simulink model "step_NL"  (R2023a)
settings: Solver=VariableStepAuto  StartTime=0.0  StopTime=70  RelTol=1e-3
values from neighbouring files (symbols this model uses):
  Ad = 60    [Script_Dirigibile.m]
  b = 20    [Script_Dirigibile.m]
  c = 12.5    [Script_Dirigibile.m]
  Cd = 0.05    [Script_Dirigibile.m]
  g = 9.81    [Script_Dirigibile.m]
  k = 15    [Script_Dirigibile.m]
  m = 1000    [Script_Dirigibile.m]
  rho_a = 1.225    [Script_Dirigibile.m]
  T_a = 288.15    [Script_Dirigibile.m]
  V = 4000    [Script_Dirigibile.m]
  x0 = [0 0 T_a]'    [Script_Dirigibile.m]
settings Model: Creator=giuco  LastModifiedBy=giuco

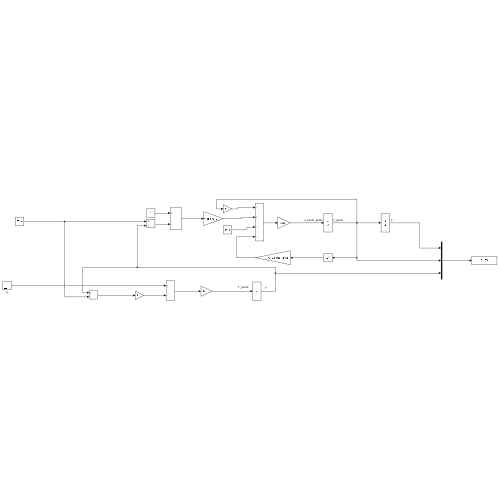
[thumbnail: Simulink's stored preview of the top-level diagram]
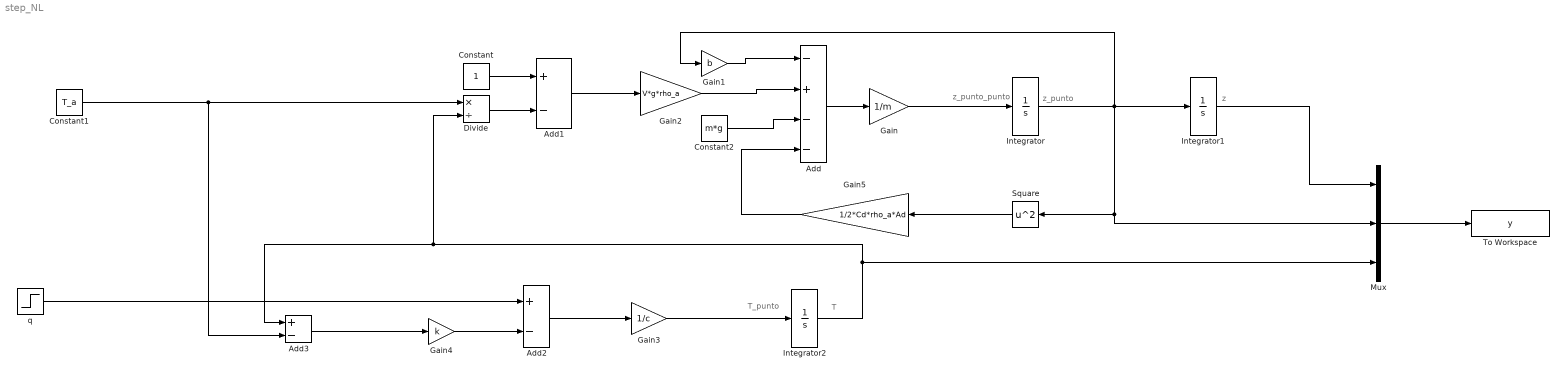
== system step_NL ==
  note: z_punto
  note: T_punto
  note: z
  note: T
  note: z_punto_punto
  Add : Sum  Inputs=-+--
  Add1 : Sum  Inputs=+-
  Add2 : Sum  Inputs=+-
  Add3 : Sum  Inputs=+-
  Constant : Constant
  Constant1 : Constant  Value=T_a
  Constant2 : Constant  Value=m*g
  Divide : Product  Inputs=*/
  Gain : Gain  Gain=1/m
  Gain1 : Gain  Gain=b
  Gain2 : Gain  Gain=V*g*rho_a
  Gain3 : Gain  Gain=1/c
  Gain4 : Gain  Gain=k
  Gain5 : Gain  Gain=1/2*Cd*rho_a*Ad
  Integrator : Integrator  InitialCondition=x0(2)
  Integrator1 : Integrator  InitialCondition=x0(1)
  Integrator2 : Integrator  InitialCondition=x0(3)
  Mux : Mux  Inputs=3
  Square : Math  Operator=square
  To Workspace : ToWorkspace  VariableName=y  SaveFormat=Timeseries  SampleTime=-1
  q : Step  Time=0  After=1500  SampleTime=0
  wires:
  Add1/1 -> Gain2/1
  q/1 -> Add2/1
  Square/1 -> Gain5/1
  Integrator1/1 -> Mux/1
  Gain2/1 -> Add/2
  Mux/1 -> To Workspace/1
  Gain3/1 -> Integrator2/1
  Constant/1 -> Add1/1
  Constant1/1 -> Add3/2, Divide/1
  Gain5/1 -> Add/4
  Add3/1 -> Gain4/1
  Integrator2/1 -> Mux/3, Add3/1, Divide/2
  Gain1/1 -> Add/1
  Divide/1 -> Add1/2
  Gain4/1 -> Add2/2
  Integrator/1 -> Square/1, Mux/2, Gain1/1, Integrator1/1
  Add2/1 -> Gain3/1
  Constant2/1 -> Add/3
  Add/1 -> Gain/1
  Gain/1 -> Integrator/1
